simulink model "bike_model_pidTuning"  (R2018b)
settings: Solver=FixedStepAuto  StartTime=0.0  StopTime=sim_time  FixedStep=Ts_IMU  MaxStep=Ts  RelTol=1e-3
values from neighbouring files (symbols this model uses):
  a_compFilter = b_compFilter - 0.77    (= 0.325)    [configuration.m]    (also in configuration_boxMovedCenter.m = 0.4964; configuration_pidTuning.m)
  b_compFilter = 1.095    [configuration.m]    (also in configuration_boxMovedCenter.m; configuration_pidTuning.m)
  b_real = 1.095    [configuration.m]    (also in configuration_boxMovedCenter.m; configuration_pidTuning.m)
  direct_control = 1    [configuration.m]    (also in configuration_boxMovedCenter.m; configuration_pidTuning.m)
  g = 9.81    [configuration.m]    (also in configuration_boxMovedCenter.m; configuration_pidTuning.m; positionEstimation.m = 9.82)
  IMU_height_real = 0.45    [configuration.m]    (also in configuration_boxMovedCenter.m; configuration_pidTuning.m)
  initial_states = [deg2rad(2) deg2rad(0) deg2rad(0)]    [configuration.m]    (also in configuration_boxMovedCenter.m = [deg2rad(5) deg2rad(-2) deg2rad(0)]; configuration_pidTuning.m = [deg2rad(0) deg2rad(0) deg2rad(0)])
  initial_x = x_ini_diff    (= 0)    [paths.m]
  initial_y = y_ini_diff    (= 0)    [paths.m]
  input_velocity = 3    [configuration.m]    (also in configuration_boxMovedCenter.m; configuration_pidTuning.m)
  K_dir = [0.2 0 0]    [tuning_pid.m]
  K_PID = K_comparison(index,:)    [tuning_pid.m]
  lambda_compFilter = deg2rad(70)    [configuration.m]    (also in configuration_boxMovedCenter.m; configuration_pidTuning.m)
  lambda_real = deg2rad(70)    [configuration.m]    (also in configuration_boxMovedCenter.m; configuration_pidTuning.m)
  look_ahead = 0    [configuration.m]    (also in configuration_boxMovedCenter.m; configuration_pidTuning.m)
  parameters_compFilter = [g h_compFilter b_compFilter a_compFilter lambda_compFilter c_compFilter]    [configuration.m]    (also in configuration_boxMovedCenter.m; configuration_pidTuning.m)
  parameters_f_b_real = [m_frame_real m_box_real h_frame_real h_box_real a_frame_real a_box_real c_frame_real c_box_real b_frame_real b_box_real l_frame_real l_box_real]    [configuration.m]    (also in configuration_boxMovedCenter.m; configuration_pidTuning.m)
  parameters_real = [g h_real b_real a_real lambda_real c_real]    [configuration.m]    (also in configuration_boxMovedCenter.m; configuration_pidTuning.m)
  path_x = [path_x1 path_x2 path_x3 path_x4 path_x5]    [paths.m]
  path_y = [path_y1 path_y2 path_y3 path_y4 path_y5]    [paths.m]
  plant_model = 1    [configuration.m]    (also in configuration_boxMovedCenter.m; configuration_pidTuning.m)
  Ts = 0.04    [configuration.m]    (also in configuration_boxMovedCenter.m; configuration_pidTuning.m; positionEstimation.m)
  Ts_IMU = 0.04    [configuration.m]    (also in configuration_boxMovedCenter.m; configuration_pidTuning.m)
undefined symbols (not defined in the file or in its folder): A, B, cumulative_dist_along_path, curvature, DiscIntNeverNeededParam, lqr_gains, sys_con, sys_dis, velocity_lqr
libraries: simulink x23, dspsigops x2
(part 2 of 3)

== system bike_model_pidTuning/Path Tracking Controller PID Tuning 2/Tuning of Direction (Heading Control) ==
  Step input : Inport
  Estimated Heading : Inport  Port=2
  Discrete-Time Integrator : DiscreteIntegrator  Commented=on  SampleTime=-1  ICPrevOutput=DiscIntNeverNeededParam  ICPrevScaledInput=DiscIntNeverNeededParam
  Gain1 : Gain  Commented=on  Gain=sin(lambda_compFilter)
  Measured Bike Angles to Global Angles : Subsystem  Commented=on
  Measured Global Angles to Global Coordinates : Subsystem  Commented=on
  PID Control Direction2 : simulink/Continuous/PID Controller  Controller=PID  Form=Parallel  TimeDomain=Discrete-time  SampleTime=Ts  IntegratorMethod=Forward Euler  FilterMethod=Forward Euler  ControllerParametersSource=internal  P=K_PID(1)  I=K_PID(2)  D=K_PID(3)  UseFilter=off  N=100  TunerSelectOption=Transfer Function Based (PID Tuner App)  InitialConditionSource=internal  InitialConditionForIntegrator=0  InitialConditionForFilter=0  DifferentiatorICPrevScaledInput=0  ExternalReset=none  TrackingMode=off  Kt=1  LimitOutput=off  UpperSaturationLimit=inf  LowerSaturationLimit=-inf  LinearizeAsGain=on  AntiWindupMode=none  Kb=1  POutMin=[]  POutMax=[]  IOutMin=[]  IOutMax=[]  DOutMin=[]  DOutMax=[]  NOutMin=[]  NOutMax=[]  SumOutMin=[]  SumOutMax=[]  SaturationOutMin=[]  SaturationOutMax=[]  PParamMin=[]  PParamMax=[]  IParamMin=[]  IParamMax=[]  DParamMin=[]  DParamMax=[]  NParamMin=[]  NParamMax=[]  KbParamMin=[]  KbParamMax=[]  KtParamMin=[]  KtParamMax=[]  KbOutMin=[]  KbOutMax=[]  KtOutMin=[]  KtOutMax=[]  IntegratorOutMin=[]  IntegratorOutMax=[]  FilterOutMin=[]  FilterOutMax=[]  SumI1OutMin=[]  SumI1OutMax=[]  SumI2OutMin=[]  SumI2OutMax=[]  SumI3OutMin=[]  SumI3OutMax=[]  SumI4OutMin=[]  SumI4OutMax=[]  SumDOutMin=[]  SumDOutMax=[]  DifferentiatorOutMin=[]  DifferentiatorOutMax=[]  FilterDiffOutCoefMin=[]  FilterDiffOutCoefMax=[]  ReciprocalOutMin=[]  ReciprocalOutMax=[]  SumDenOutMin=[]  SumDenOutMax=[]  SumNumOutMin=[]  SumNumOutMax=[]  DivideOutMin=[]  DivideOutMax=[]  IntegratorContinuousStateAttributes=''  IntegratorStateMustResolveToSignalObject=off  IntegratorRTWStateStorageClass=Auto  FilterContinuousStateAttributes=''  FilterStateMustResolveToSignalObject=off  FilterRTWStateStorageClass=Auto  ParallelPVariant=InternalParameters  IdealPVariant=Disabled  IVariant=InternalParameters  DVariant=InternalParameters  IntegratorVariant=Discrete  SatVariant=Disabled  AWVariant=Passthrough  PCopyVariant=Disabled  TRVariant=Disabled  FdbkBlocksVariant=Forward  IdealPFdbkVariant=Disabled  SatFdbkVariant=Disabled  DerivativeFilterVariant=Differentiator  NVariant=Passthrough  NCopyVariant=Disabled_SignalSpec  FilterICVariant=InternalICsDifferentiator  IntegratorICVariant=InternalICs  ExternalResetVariant=Disabled  TRSumVariant=Passthrough  SumFdbkVariant=Disabled  SumVariant=Sum_PID
  Psi to Delta : Subsystem  Commented=on
  Sum : Sum  Commented=on  Inputs=++|
  Sum4 : Sum  Inputs=+--
  To Workspace5 : ToWorkspace  Commented=on  VariableName=pos_vel_int1  SaveFormat=Timeseries  SampleTime=-1
  Steering Reference : Outport
  Controlled Output : Outport  Port=2
  wires:
  Estimated Heading/1 -> Controlled Output/1, Sum4/3
  Sum4/1 -> PID Control Direction2/1  "Delta Reference = Psi Sigma - Nu"
  Step input/1 -> Sum4/1
  PID Control Direction2/1 -> Steering Reference/1
  Measured Bike Angles to Global Angles/1(Psi) -> Sum/2, Measured Global Angles to Global Coordinates/2(Psi)
  ? -> Gain1/1
  Measured Global Angles to Global Coordinates/1("Velocity (Xdot, Ydot)") -> Discrete-Time Integrator/1
  Gain1/1 -> Measured Bike Angles to Global Angles/2(Measured Steering Angle)
  Sum/1 -> ?
  ? -> Measured Bike Angles to Global Angles/1(Velocity), Measured Global Angles to Global Coordinates/1(Velocity)
  Measured Bike Angles to Global Angles/2(Beta) -> Measured Global Angles to Global Coordinates/3(Beta), Sum/1
  Discrete-Time Integrator/1 -> To Workspace5/1

== system bike_model_pidTuning/Path Tracking Controller PID Tuning 2/Tuning of Direction (Heading Control)2 ==
  Step input : Inport
  Measured Steering : Inport  Port=2
  PID Control Direction2 : simulink/Continuous/PID Controller  Controller=PI  Form=Parallel  TimeDomain=Discrete-time  SampleTime=Ts  IntegratorMethod=Forward Euler  FilterMethod=Forward Euler  ControllerParametersSource=internal  P=0.578359413467721  I=0.617399561418389  D=0  UseFilter=on  N=100  TunerSelectOption=Transfer Function Based (PID Tuner App)  InitialConditionSource=internal  InitialConditionForIntegrator=0  InitialConditionForFilter=0  DifferentiatorICPrevScaledInput=0  ExternalReset=none  TrackingMode=off  Kt=1  LimitOutput=off  UpperSaturationLimit=inf  LowerSaturationLimit=-inf  LinearizeAsGain=on  AntiWindupMode=none  Kb=1  POutMin=[]  POutMax=[]  IOutMin=[]  IOutMax=[]  DOutMin=[]  DOutMax=[]  NOutMin=[]  NOutMax=[]  SumOutMin=[]  SumOutMax=[]  SaturationOutMin=[]  SaturationOutMax=[]  PParamMin=[]  PParamMax=[]  IParamMin=[]  IParamMax=[]  DParamMin=[]  DParamMax=[]  NParamMin=[]  NParamMax=[]  KbParamMin=[]  KbParamMax=[]  KtParamMin=[]  KtParamMax=[]  KbOutMin=[]  KbOutMax=[]  KtOutMin=[]  KtOutMax=[]  IntegratorOutMin=[]  IntegratorOutMax=[]  FilterOutMin=[]  FilterOutMax=[]  SumI1OutMin=[]  SumI1OutMax=[]  SumI2OutMin=[]  SumI2OutMax=[]  SumI3OutMin=[]  SumI3OutMax=[]  SumI4OutMin=[]  SumI4OutMax=[]  SumDOutMin=[]  SumDOutMax=[]  DifferentiatorOutMin=[]  DifferentiatorOutMax=[]  FilterDiffOutCoefMin=[]  FilterDiffOutCoefMax=[]  ReciprocalOutMin=[]  ReciprocalOutMax=[]  SumDenOutMin=[]  SumDenOutMax=[]  SumNumOutMin=[]  SumNumOutMax=[]  DivideOutMin=[]  DivideOutMax=[]  IntegratorContinuousStateAttributes=''  IntegratorStateMustResolveToSignalObject=off  IntegratorRTWStateStorageClass=Auto  FilterContinuousStateAttributes=''  FilterStateMustResolveToSignalObject=off  FilterRTWStateStorageClass=Auto  ParallelPVariant=InternalParameters  IdealPVariant=Disabled  IVariant=InternalParameters  DVariant=Disabled  IntegratorVariant=Discrete  SatVariant=Disabled  AWVariant=Passthrough  PCopyVariant=Disabled  TRVariant=Disabled  FdbkBlocksVariant=Forward  IdealPFdbkVariant=Disabled  SatFdbkVariant=Disabled  DerivativeFilterVariant=Disabled  NVariant=Disabled  NCopyVariant=Disabled_SignalSpec  FilterICVariant=Disabled  IntegratorICVariant=InternalICs  ExternalResetVariant=Disabled  TRSumVariant=Passthrough  SumFdbkVariant=Disabled  SumVariant=Sum_PI
  Sum4 : Sum  Inputs=+--
  Transfer Fcn : TransferFcn  Numerator=[1 0]  Denominator=[a_compFilter/b_compFilter input_velocity/a_compFilter]
  Steering Reference : Outport
  Controlled Output : Outport  Port=2
  wires:
  Step input/1 -> Transfer Fcn/1
  PID Control Direction2/1 -> Steering Reference/1
  Measured Steering/1 -> Controlled Output/1, Sum4/3
  Transfer Fcn/1 -> Sum4/1
  Sum4/1 -> PID Control Direction2/1

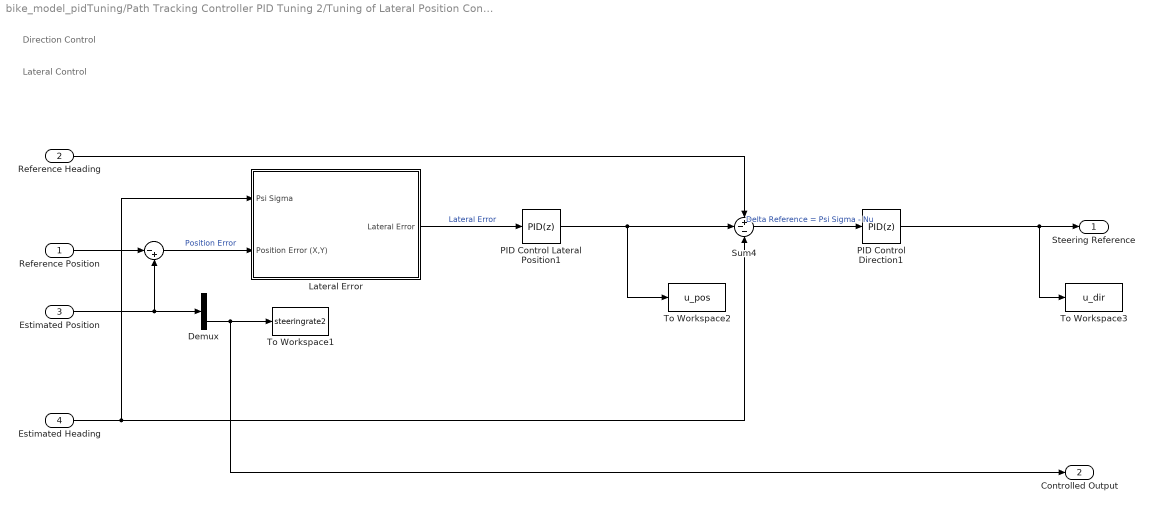
== system bike_model_pidTuning/Path Tracking Controller PID Tuning 2/Tuning of Lateral Position Control ==
  note: Direction Control
  note: Lateral Control
  Reference Position : Inport
  Reference Heading : Inport  Port=2
  Estimated Position : Inport  Port=3
  Estimated Heading : Inport  Port=4
  " " : Sum  Inputs=|-+
  Demux : Demux  Outputs=2
  Lateral Error : Subsystem  SystemSampleTime=Ts
  PID Control Lateral Position1 : simulink/Continuous/PID Controller  Controller=PID  Form=Parallel  TimeDomain=Discrete-time  SampleTime=Ts  IntegratorMethod=Forward Euler  FilterMethod=Forward Euler  ControllerParametersSource=internal  P=K_PID(1)  I=K_PID(2)  D=K_PID(3)  UseFilter=off  N=38.085941813801  TunerSelectOption=Transfer Function Based (PID Tuner App)  InitialConditionSource=internal  InitialConditionForIntegrator=0  InitialConditionForFilter=0  DifferentiatorICPrevScaledInput=0  ExternalReset=none  TrackingMode=off  Kt=1  LimitOutput=off  UpperSaturationLimit=inf  LowerSaturationLimit=-inf  LinearizeAsGain=on  AntiWindupMode=none  Kb=1  POutMin=[]  POutMax=[]  IOutMin=[]  IOutMax=[]  DOutMin=[]  DOutMax=[]  NOutMin=[]  NOutMax=[]  SumOutMin=[]  SumOutMax=[]  SaturationOutMin=[]  SaturationOutMax=[]  PParamMin=[]  PParamMax=[]  IParamMin=[]  IParamMax=[]  DParamMin=[]  DParamMax=[]  NParamMin=[]  NParamMax=[]  KbParamMin=[]  KbParamMax=[]  KtParamMin=[]  KtParamMax=[]  KbOutMin=[]  KbOutMax=[]  KtOutMin=[]  KtOutMax=[]  IntegratorOutMin=[]  IntegratorOutMax=[]  FilterOutMin=[]  FilterOutMax=[]  SumI1OutMin=[]  SumI1OutMax=[]  SumI2OutMin=[]  SumI2OutMax=[]  SumI3OutMin=[]  SumI3OutMax=[]  SumI4OutMin=[]  SumI4OutMax=[]  SumDOutMin=[]  SumDOutMax=[]  DifferentiatorOutMin=[]  DifferentiatorOutMax=[]  FilterDiffOutCoefMin=[]  FilterDiffOutCoefMax=[]  ReciprocalOutMin=[]  ReciprocalOutMax=[]  SumDenOutMin=[]  SumDenOutMax=[]  SumNumOutMin=[]  SumNumOutMax=[]  DivideOutMin=[]  DivideOutMax=[]  IntegratorContinuousStateAttributes=''  IntegratorStateMustResolveToSignalObject=off  IntegratorRTWStateStorageClass=Auto  FilterContinuousStateAttributes=''  FilterStateMustResolveToSignalObject=off  FilterRTWStateStorageClass=Auto  ParallelPVariant=InternalParameters  IdealPVariant=Disabled  IVariant=InternalParameters  DVariant=InternalParameters  IntegratorVariant=Discrete  SatVariant=Disabled  AWVariant=Passthrough  PCopyVariant=Disabled  TRVariant=Disabled  FdbkBlocksVariant=Forward  IdealPFdbkVariant=Disabled  SatFdbkVariant=Disabled  DerivativeFilterVariant=Differentiator  NVariant=Passthrough  NCopyVariant=Disabled_SignalSpec  FilterICVariant=InternalICsDifferentiator  IntegratorICVariant=InternalICs  ExternalResetVariant=Disabled  TRSumVariant=Passthrough  SumFdbkVariant=Disabled  SumVariant=Sum_PID
  PID Control Direction1 : simulink/Continuous/PID Controller  Controller=PID  Form=Parallel  TimeDomain=Discrete-time  SampleTime=Ts  IntegratorMethod=Forward Euler  FilterMethod=Forward Euler  ControllerParametersSource=internal  P=K_dir(1)  I=K_dir(2)  D=K_dir(3)  UseFilter=off  N=100  TunerSelectOption=Transfer Function Based (PID Tuner App)  InitialConditionSource=internal  InitialConditionForIntegrator=0  InitialConditionForFilter=0  DifferentiatorICPrevScaledInput=0  ExternalReset=none  TrackingMode=off  Kt=1  LimitOutput=off  UpperSaturationLimit=inf  LowerSaturationLimit=-inf  LinearizeAsGain=on  AntiWindupMode=none  Kb=1  POutMin=[]  POutMax=[]  IOutMin=[]  IOutMax=[]  DOutMin=[]  DOutMax=[]  NOutMin=[]  NOutMax=[]  SumOutMin=[]  SumOutMax=[]  SaturationOutMin=[]  SaturationOutMax=[]  PParamMin=[]  PParamMax=[]  IParamMin=[]  IParamMax=[]  DParamMin=[]  DParamMax=[]  NParamMin=[]  NParamMax=[]  KbParamMin=[]  KbParamMax=[]  KtParamMin=[]  KtParamMax=[]  KbOutMin=[]  KbOutMax=[]  KtOutMin=[]  KtOutMax=[]  IntegratorOutMin=[]  IntegratorOutMax=[]  FilterOutMin=[]  FilterOutMax=[]  SumI1OutMin=[]  SumI1OutMax=[]  SumI2OutMin=[]  SumI2OutMax=[]  SumI3OutMin=[]  SumI3OutMax=[]  SumI4OutMin=[]  SumI4OutMax=[]  SumDOutMin=[]  SumDOutMax=[]  DifferentiatorOutMin=[]  DifferentiatorOutMax=[]  FilterDiffOutCoefMin=[]  FilterDiffOutCoefMax=[]  ReciprocalOutMin=[]  ReciprocalOutMax=[]  SumDenOutMin=[]  SumDenOutMax=[]  SumNumOutMin=[]  SumNumOutMax=[]  DivideOutMin=[]  DivideOutMax=[]  IntegratorContinuousStateAttributes=''  IntegratorStateMustResolveToSignalObject=off  IntegratorRTWStateStorageClass=Auto  FilterContinuousStateAttributes=''  FilterStateMustResolveToSignalObject=off  FilterRTWStateStorageClass=Auto  ParallelPVariant=InternalParameters  IdealPVariant=Disabled  IVariant=InternalParameters  DVariant=InternalParameters  IntegratorVariant=Discrete  SatVariant=Disabled  AWVariant=Passthrough  PCopyVariant=Disabled  TRVariant=Disabled  FdbkBlocksVariant=Forward  IdealPFdbkVariant=Disabled  SatFdbkVariant=Disabled  DerivativeFilterVariant=Differentiator  NVariant=Passthrough  NCopyVariant=Disabled_SignalSpec  FilterICVariant=InternalICsDifferentiator  IntegratorICVariant=InternalICs  ExternalResetVariant=Disabled  TRSumVariant=Passthrough  SumFdbkVariant=Disabled  SumVariant=Sum_PID
  Sum4 : Sum  Inputs=+--
  To Workspace1 : ToWorkspace  VariableName=steeringrate2  SaveFormat=Timeseries  SampleTime=Ts
  To Workspace2 : ToWorkspace  VariableName=u_pos  SaveFormat=Timeseries  SampleTime=Ts
  To Workspace3 : ToWorkspace  VariableName=u_dir  SaveFormat=Timeseries  SampleTime=Ts
  Steering Reference : Outport
  Controlled Output : Outport  Port=2
  wires:
  PID Control Lateral Position1/1 -> To Workspace2/1, Sum4/2
  Reference Heading/1 -> Sum4/1
  Lateral Error/1(Lateral Error) -> PID Control Lateral Position1/1  "Lateral Error"
  Reference Position/1 -> " "/1
  Estimated Heading/1 -> Lateral Error/1(Psi Sigma), Sum4/3
  " "/1 -> Lateral Error/2(Position Error (X,Y))  "Position Error"
  Sum4/1 -> PID Control Direction1/1  "Delta Reference = Psi Sigma - Nu"
  Demux/2 -> Controlled Output/1, To Workspace1/1
  PID Control Direction1/1 -> To Workspace3/1, Steering Reference/1
  Estimated Position/1 -> " "/2, Demux/1

== system bike_model_pidTuning/Path Tracking Controller PID Tuning 2/Tuning of Lateral Position Control1 ==
  note: Direction Control
  note: Lateral Control
  Reference Position : Inport
  Reference Heading : Inport  Port=2
  Estimated Position : Inport  Port=3
  Estimated Heading : Inport  Port=4
  " " : Sum  Inputs=|-+
  Demux : Demux  Outputs=2
  Lateral Error : Subsystem  SystemSampleTime=Ts
  PID Control Lateral Position : simulink/Continuous/PID Controller  Controller=PID  Form=Parallel  TimeDomain=Discrete-time  SampleTime=Ts  IntegratorMethod=Forward Euler  FilterMethod=Forward Euler  ControllerParametersSource=internal  P=0.0553  I=0.000972  D=0.699  UseFilter=on  N=100  TunerSelectOption=Transfer Function Based (PID Tuner App)  InitialConditionSource=internal  InitialConditionForIntegrator=0  InitialConditionForFilter=0  DifferentiatorICPrevScaledInput=0  ExternalReset=none  TrackingMode=off  Kt=1  LimitOutput=off  UpperSaturationLimit=inf  LowerSaturationLimit=-inf  LinearizeAsGain=on  AntiWindupMode=none  Kb=1  POutMin=[]  POutMax=[]  IOutMin=[]  IOutMax=[]  DOutMin=[]  DOutMax=[]  NOutMin=[]  NOutMax=[]  SumOutMin=[]  SumOutMax=[]  SaturationOutMin=[]  SaturationOutMax=[]  PParamMin=[]  PParamMax=[]  IParamMin=[]  IParamMax=[]  DParamMin=[]  DParamMax=[]  NParamMin=[]  NParamMax=[]  KbParamMin=[]  KbParamMax=[]  KtParamMin=[]  KtParamMax=[]  KbOutMin=[]  KbOutMax=[]  KtOutMin=[]  KtOutMax=[]  IntegratorOutMin=[]  IntegratorOutMax=[]  FilterOutMin=[]  FilterOutMax=[]  SumI1OutMin=[]  SumI1OutMax=[]  SumI2OutMin=[]  SumI2OutMax=[]  SumI3OutMin=[]  SumI3OutMax=[]  SumI4OutMin=[]  SumI4OutMax=[]  SumDOutMin=[]  SumDOutMax=[]  DifferentiatorOutMin=[]  DifferentiatorOutMax=[]  FilterDiffOutCoefMin=[]  FilterDiffOutCoefMax=[]  ReciprocalOutMin=[]  ReciprocalOutMax=[]  SumDenOutMin=[]  SumDenOutMax=[]  SumNumOutMin=[]  SumNumOutMax=[]  DivideOutMin=[]  DivideOutMax=[]  IntegratorContinuousStateAttributes=''  IntegratorStateMustResolveToSignalObject=off  IntegratorRTWStateStorageClass=Auto  FilterContinuousStateAttributes=''  FilterStateMustResolveToSignalObject=off  FilterRTWStateStorageClass=Auto  ParallelPVariant=InternalParameters  IdealPVariant=Disabled  IVariant=InternalParameters  DVariant=InternalParameters  IntegratorVariant=Discrete  SatVariant=Disabled  AWVariant=Passthrough  PCopyVariant=Disabled  TRVariant=Disabled  FdbkBlocksVariant=Forward  IdealPFdbkVariant=Disabled  SatFdbkVariant=Disabled  DerivativeFilterVariant=ForwardEulerFilter  NVariant=InternalParameters  NCopyVariant=Disabled  FilterICVariant=InternalICsFilter  IntegratorICVariant=InternalICs  ExternalResetVariant=Disabled  TRSumVariant=Passthrough  SumFdbkVariant=Disabled  SumVariant=Sum_PID
  PID Control Direction2 : simulink/Continuous/PID Controller  Controller=PI  Form=Parallel  TimeDomain=Discrete-time  SampleTime=Ts  IntegratorMethod=Forward Euler  FilterMethod=Forward Euler  ControllerParametersSource=internal  P=0.578359413467721  I=0.617399561418389  D=0  UseFilter=on  N=100  TunerSelectOption=Transfer Function Based (PID Tuner App)  InitialConditionSource=internal  InitialConditionForIntegrator=0  InitialConditionForFilter=0  DifferentiatorICPrevScaledInput=0  ExternalReset=none  TrackingMode=off  Kt=1  LimitOutput=off  UpperSaturationLimit=inf  LowerSaturationLimit=-inf  LinearizeAsGain=on  AntiWindupMode=none  Kb=1  POutMin=[]  POutMax=[]  IOutMin=[]  IOutMax=[]  DOutMin=[]  DOutMax=[]  NOutMin=[]  NOutMax=[]  SumOutMin=[]  SumOutMax=[]  SaturationOutMin=[]  SaturationOutMax=[]  PParamMin=[]  PParamMax=[]  IParamMin=[]  IParamMax=[]  DParamMin=[]  DParamMax=[]  NParamMin=[]  NParamMax=[]  KbParamMin=[]  KbParamMax=[]  KtParamMin=[]  KtParamMax=[]  KbOutMin=[]  KbOutMax=[]  KtOutMin=[]  KtOutMax=[]  IntegratorOutMin=[]  IntegratorOutMax=[]  FilterOutMin=[]  FilterOutMax=[]  SumI1OutMin=[]  SumI1OutMax=[]  SumI2OutMin=[]  SumI2OutMax=[]  SumI3OutMin=[]  SumI3OutMax=[]  SumI4OutMin=[]  SumI4OutMax=[]  SumDOutMin=[]  SumDOutMax=[]  DifferentiatorOutMin=[]  DifferentiatorOutMax=[]  FilterDiffOutCoefMin=[]  FilterDiffOutCoefMax=[]  ReciprocalOutMin=[]  ReciprocalOutMax=[]  SumDenOutMin=[]  SumDenOutMax=[]  SumNumOutMin=[]  SumNumOutMax=[]  DivideOutMin=[]  DivideOutMax=[]  IntegratorContinuousStateAttributes=''  IntegratorStateMustResolveToSignalObject=off  IntegratorRTWStateStorageClass=Auto  FilterContinuousStateAttributes=''  FilterStateMustResolveToSignalObject=off  FilterRTWStateStorageClass=Auto  ParallelPVariant=InternalParameters  IdealPVariant=Disabled  IVariant=InternalParameters  DVariant=Disabled  IntegratorVariant=Discrete  SatVariant=Disabled  AWVariant=Passthrough  PCopyVariant=Disabled  TRVariant=Disabled  FdbkBlocksVariant=Forward  IdealPFdbkVariant=Disabled  SatFdbkVariant=Disabled  DerivativeFilterVariant=Disabled  NVariant=Disabled  NCopyVariant=Disabled_SignalSpec  FilterICVariant=Disabled  IntegratorICVariant=InternalICs  ExternalResetVariant=Disabled  TRSumVariant=Passthrough  SumFdbkVariant=Disabled  SumVariant=Sum_PI
  Sum4 : Sum  Inputs=+--
  Transfer Fcn : TransferFcn  Numerator=[1 0]  Denominator=[a_compFilter/b_compFilter input_velocity/a_compFilter]
  Steering Reference : Outport
  Controlled Output : Outport  Port=2
  wires:
  Reference Heading/1 -> Transfer Fcn/1, Lateral Error/1(Psi Sigma)
  Lateral Error/1(Lateral Error) -> PID Control Lateral Position/1  "Lateral Error"
  Reference Position/1 -> " "/1
  Estimated Heading/1 -> Sum4/3
  " "/1 -> Lateral Error/2(Position Error (X,Y))  "Position Error"
  Sum4/1 -> PID Control Direction2/1  "Delta Reference = Psi Sigma - Nu"
  Demux/2 -> Controlled Output/1
  PID Control Direction2/1 -> Steering Reference/1
  Estimated Position/1 -> " "/2, Demux/1
  Transfer Fcn/1 -> Sum4/1
  PID Control Lateral Position/1 -> Sum4/2

== system bike_model_pidTuning/Path Tracking Controller PID Tuning1/Step response of the system ==
  Step input : Inport
  Measured Steering Angle : Inport  Port=2
  Gain : Gain  Gain=2/3
  Steering Reference : Outport
  Controlled Output : Outport  Port=2
  wires:
  Step input/1 -> Gain/1
  Measured Steering Angle/1 -> Controlled Output/1
  Gain/1 -> Steering Reference/1

== system bike_model_pidTuning/Path Tracking Controller PID Tuning1/Tuning of Direction (Heading Control) ==
  Step input : Inport
  Estimated Heading : Inport  Port=2
  Measured Steering Angle : Inport  Port=3
  Gain1 : Gain  Gain=1%sin(lambda_real)
  PID Control Direction : simulink/Continuous/PID Controller  Controller=PI  Form=Parallel  TimeDomain=Discrete-time  SampleTime=Ts  IntegratorMethod=Forward Euler  FilterMethod=Forward Euler  ControllerParametersSource=internal  P=0.0712859744206787*2  I=0.000227125326188444/2  D=0  UseFilter=on  N=100  TunerSelectOption=Transfer Function Based (PID Tuner App)  InitialConditionSource=internal  InitialConditionForIntegrator=0  InitialConditionForFilter=0  DifferentiatorICPrevScaledInput=0  ExternalReset=none  TrackingMode=off  Kt=1  LimitOutput=off  UpperSaturationLimit=inf  LowerSaturationLimit=-inf  LinearizeAsGain=on  AntiWindupMode=none  Kb=1  POutMin=[]  POutMax=[]  IOutMin=[]  IOutMax=[]  DOutMin=[]  DOutMax=[]  NOutMin=[]  NOutMax=[]  SumOutMin=[]  SumOutMax=[]  SaturationOutMin=[]  SaturationOutMax=[]  PParamMin=[]  PParamMax=[]  IParamMin=[]  IParamMax=[]  DParamMin=[]  DParamMax=[]  NParamMin=[]  NParamMax=[]  KbParamMin=[]  KbParamMax=[]  KtParamMin=[]  KtParamMax=[]  KbOutMin=[]  KbOutMax=[]  KtOutMin=[]  KtOutMax=[]  IntegratorOutMin=[]  IntegratorOutMax=[]  FilterOutMin=[]  FilterOutMax=[]  SumI1OutMin=[]  SumI1OutMax=[]  SumI2OutMin=[]  SumI2OutMax=[]  SumI3OutMin=[]  SumI3OutMax=[]  SumI4OutMin=[]  SumI4OutMax=[]  SumDOutMin=[]  SumDOutMax=[]  DifferentiatorOutMin=[]  DifferentiatorOutMax=[]  FilterDiffOutCoefMin=[]  FilterDiffOutCoefMax=[]  ReciprocalOutMin=[]  ReciprocalOutMax=[]  SumDenOutMin=[]  SumDenOutMax=[]  SumNumOutMin=[]  SumNumOutMax=[]  DivideOutMin=[]  DivideOutMax=[]  IntegratorContinuousStateAttributes=''  IntegratorStateMustResolveToSignalObject=off  IntegratorRTWStateStorageClass=Auto  FilterContinuousStateAttributes=''  FilterStateMustResolveToSignalObject=off  FilterRTWStateStorageClass=Auto  ParallelPVariant=InternalParameters  IdealPVariant=Disabled  IVariant=InternalParameters  DVariant=Disabled  IntegratorVariant=Discrete  SatVariant=Disabled  AWVariant=Passthrough  PCopyVariant=Disabled  TRVariant=Disabled  FdbkBlocksVariant=Forward  IdealPFdbkVariant=Disabled  SatFdbkVariant=Disabled  DerivativeFilterVariant=Disabled  NVariant=Disabled  NCopyVariant=Disabled_SignalSpec  FilterICVariant=Disabled  IntegratorICVariant=InternalICs  ExternalResetVariant=Disabled  TRSumVariant=Passthrough  SumFdbkVariant=Disabled  SumVariant=Sum_PI
  PID Control Steering : simulink/Continuous/PID Controller  Controller=PI  Form=Parallel  TimeDomain=Discrete-time  SampleTime=Ts  IntegratorMethod=Forward Euler  FilterMethod=Forward Euler  ControllerParametersSource=internal  P=0.219020351848633  I=0.4510120195392  D=0  UseFilter=on  N=100  TunerSelectOption=Transfer Function Based (PID Tuner App)  InitialConditionSource=internal  InitialConditionForIntegrator=0  InitialConditionForFilter=0  DifferentiatorICPrevScaledInput=0  ExternalReset=none  TrackingMode=off  Kt=1  LimitOutput=off  UpperSaturationLimit=inf  LowerSaturationLimit=-inf  LinearizeAsGain=on  AntiWindupMode=none  Kb=1  POutMin=[]  POutMax=[]  IOutMin=[]  IOutMax=[]  DOutMin=[]  DOutMax=[]  NOutMin=[]  NOutMax=[]  SumOutMin=[]  SumOutMax=[]  SaturationOutMin=[]  SaturationOutMax=[]  PParamMin=[]  PParamMax=[]  IParamMin=[]  IParamMax=[]  DParamMin=[]  DParamMax=[]  NParamMin=[]  NParamMax=[]  KbParamMin=[]  KbParamMax=[]  KtParamMin=[]  KtParamMax=[]  KbOutMin=[]  KbOutMax=[]  KtOutMin=[]  KtOutMax=[]  IntegratorOutMin=[]  IntegratorOutMax=[]  FilterOutMin=[]  FilterOutMax=[]  SumI1OutMin=[]  SumI1OutMax=[]  SumI2OutMin=[]  SumI2OutMax=[]  SumI3OutMin=[]  SumI3OutMax=[]  SumI4OutMin=[]  SumI4OutMax=[]  SumDOutMin=[]  SumDOutMax=[]  DifferentiatorOutMin=[]  DifferentiatorOutMax=[]  FilterDiffOutCoefMin=[]  FilterDiffOutCoefMax=[]  ReciprocalOutMin=[]  ReciprocalOutMax=[]  SumDenOutMin=[]  SumDenOutMax=[]  SumNumOutMin=[]  SumNumOutMax=[]  DivideOutMin=[]  DivideOutMax=[]  IntegratorContinuousStateAttributes=''  IntegratorStateMustResolveToSignalObject=off  IntegratorRTWStateStorageClass=Auto  FilterContinuousStateAttributes=''  FilterStateMustResolveToSignalObject=off  FilterRTWStateStorageClass=Auto  ParallelPVariant=InternalParameters  IdealPVariant=Disabled  IVariant=InternalParameters  DVariant=Disabled  IntegratorVariant=Discrete  SatVariant=Disabled  AWVariant=Passthrough  PCopyVariant=Disabled  TRVariant=Disabled  FdbkBlocksVariant=Forward  IdealPFdbkVariant=Disabled  SatFdbkVariant=Disabled  DerivativeFilterVariant=Disabled  NVariant=Disabled  NCopyVariant=Disabled_SignalSpec  FilterICVariant=Disabled  IntegratorICVariant=InternalICs  ExternalResetVariant=Disabled  TRSumVariant=Passthrough  SumFdbkVariant=Disabled  SumVariant=Sum_PI
  Sum1 : Sum  Inputs=|+-
  Sum4 : Sum  Inputs=+--
  Steering Reference : Outport
  Controlled Output : Outport  Port=2
  wires:
  Sum1/1 -> PID Control Steering/1  "Delta Error"
  PID Control Direction/1 -> Sum1/1
  Estimated Heading/1 -> Sum4/3, Controlled Output/1
  Sum4/1 -> PID Control Direction/1  "Delta Reference = Psi Sigma - Nu"
  Step input/1 -> Sum4/1
  Measured Steering Angle/1 -> Gain1/1
  Gain1/1 -> Sum1/2
  PID Control Steering/1 -> Steering Reference/1

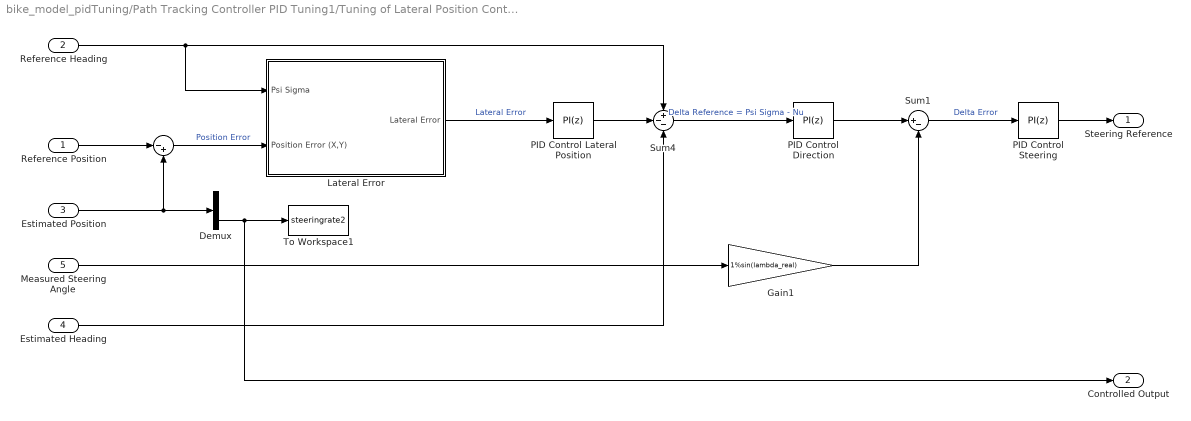
== system bike_model_pidTuning/Path Tracking Controller PID Tuning1/Tuning of Lateral Position Control ==
  Reference Position : Inport
  Reference Heading : Inport  Port=2
  Estimated Position : Inport  Port=3
  Estimated Heading : Inport  Port=4
  Measured Steering Angle : Inport  Port=5
  " " : Sum  Inputs=|-+
  Demux : Demux  Outputs=2
  Gain1 : Gain  Gain=1%sin(lambda_real)
  Lateral Error : Subsystem  SystemSampleTime=Ts
  PID Control Lateral Position : simulink/Continuous/PID Controller  Controller=PI  Form=Parallel  TimeDomain=Discrete-time  SampleTime=Ts  IntegratorMethod=Forward Euler  FilterMethod=Forward Euler  ControllerParametersSource=internal  P=0.0465435246389258  I=0.000115580509653549  D=0  UseFilter=on  N=100  TunerSelectOption=Transfer Function Based (PID Tuner App)  InitialConditionSource=internal  InitialConditionForIntegrator=0  InitialConditionForFilter=0  DifferentiatorICPrevScaledInput=0  ExternalReset=none  TrackingMode=off  Kt=1  LimitOutput=off  UpperSaturationLimit=inf  LowerSaturationLimit=-inf  LinearizeAsGain=on  AntiWindupMode=none  Kb=1  POutMin=[]  POutMax=[]  IOutMin=[]  IOutMax=[]  DOutMin=[]  DOutMax=[]  NOutMin=[]  NOutMax=[]  SumOutMin=[]  SumOutMax=[]  SaturationOutMin=[]  SaturationOutMax=[]  PParamMin=[]  PParamMax=[]  IParamMin=[]  IParamMax=[]  DParamMin=[]  DParamMax=[]  NParamMin=[]  NParamMax=[]  KbParamMin=[]  KbParamMax=[]  KtParamMin=[]  KtParamMax=[]  KbOutMin=[]  KbOutMax=[]  KtOutMin=[]  KtOutMax=[]  IntegratorOutMin=[]  IntegratorOutMax=[]  FilterOutMin=[]  FilterOutMax=[]  SumI1OutMin=[]  SumI1OutMax=[]  SumI2OutMin=[]  SumI2OutMax=[]  SumI3OutMin=[]  SumI3OutMax=[]  SumI4OutMin=[]  SumI4OutMax=[]  SumDOutMin=[]  SumDOutMax=[]  DifferentiatorOutMin=[]  DifferentiatorOutMax=[]  FilterDiffOutCoefMin=[]  FilterDiffOutCoefMax=[]  ReciprocalOutMin=[]  ReciprocalOutMax=[]  SumDenOutMin=[]  SumDenOutMax=[]  SumNumOutMin=[]  SumNumOutMax=[]  DivideOutMin=[]  DivideOutMax=[]  IntegratorContinuousStateAttributes=''  IntegratorStateMustResolveToSignalObject=off  IntegratorRTWStateStorageClass=Auto  FilterContinuousStateAttributes=''  FilterStateMustResolveToSignalObject=off  FilterRTWStateStorageClass=Auto  ParallelPVariant=InternalParameters  IdealPVariant=Disabled  IVariant=InternalParameters  DVariant=Disabled  IntegratorVariant=Discrete  SatVariant=Disabled  AWVariant=Passthrough  PCopyVariant=Disabled  TRVariant=Disabled  FdbkBlocksVariant=Forward  IdealPFdbkVariant=Disabled  SatFdbkVariant=Disabled  DerivativeFilterVariant=Disabled  NVariant=Disabled  NCopyVariant=Disabled_SignalSpec  FilterICVariant=Disabled  IntegratorICVariant=InternalICs  ExternalResetVariant=Disabled  TRSumVariant=Passthrough  SumFdbkVariant=Disabled  SumVariant=Sum_PI
  PID Control Direction : simulink/Continuous/PID Controller  Controller=PI  Form=Parallel  TimeDomain=Discrete-time  SampleTime=Ts  IntegratorMethod=Forward Euler  FilterMethod=Forward Euler  ControllerParametersSource=internal  P=0.126067479140802  I=0.000739995118675849  D=0  UseFilter=on  N=100  TunerSelectOption=Transfer Function Based (PID Tuner App)  InitialConditionSource=internal  InitialConditionForIntegrator=0  InitialConditionForFilter=0  DifferentiatorICPrevScaledInput=0  ExternalReset=none  TrackingMode=off  Kt=1  LimitOutput=off  UpperSaturationLimit=inf  LowerSaturationLimit=-inf  LinearizeAsGain=on  AntiWindupMode=none  Kb=1  POutMin=[]  POutMax=[]  IOutMin=[]  IOutMax=[]  DOutMin=[]  DOutMax=[]  NOutMin=[]  NOutMax=[]  SumOutMin=[]  SumOutMax=[]  SaturationOutMin=[]  SaturationOutMax=[]  PParamMin=[]  PParamMax=[]  IParamMin=[]  IParamMax=[]  DParamMin=[]  DParamMax=[]  NParamMin=[]  NParamMax=[]  KbParamMin=[]  KbParamMax=[]  KtParamMin=[]  KtParamMax=[]  KbOutMin=[]  KbOutMax=[]  KtOutMin=[]  KtOutMax=[]  IntegratorOutMin=[]  IntegratorOutMax=[]  FilterOutMin=[]  FilterOutMax=[]  SumI1OutMin=[]  SumI1OutMax=[]  SumI2OutMin=[]  SumI2OutMax=[]  SumI3OutMin=[]  SumI3OutMax=[]  SumI4OutMin=[]  SumI4OutMax=[]  SumDOutMin=[]  SumDOutMax=[]  DifferentiatorOutMin=[]  DifferentiatorOutMax=[]  FilterDiffOutCoefMin=[]  FilterDiffOutCoefMax=[]  ReciprocalOutMin=[]  ReciprocalOutMax=[]  SumDenOutMin=[]  SumDenOutMax=[]  SumNumOutMin=[]  SumNumOutMax=[]  DivideOutMin=[]  DivideOutMax=[]  IntegratorContinuousStateAttributes=''  IntegratorStateMustResolveToSignalObject=off  IntegratorRTWStateStorageClass=Auto  FilterContinuousStateAttributes=''  FilterStateMustResolveToSignalObject=off  FilterRTWStateStorageClass=Auto  ParallelPVariant=InternalParameters  IdealPVariant=Disabled  IVariant=InternalParameters  DVariant=Disabled  IntegratorVariant=Discrete  SatVariant=Disabled  AWVariant=Passthrough  PCopyVariant=Disabled  TRVariant=Disabled  FdbkBlocksVariant=Forward  IdealPFdbkVariant=Disabled  SatFdbkVariant=Disabled  DerivativeFilterVariant=Disabled  NVariant=Disabled  NCopyVariant=Disabled_SignalSpec  FilterICVariant=Disabled  IntegratorICVariant=InternalICs  ExternalResetVariant=Disabled  TRSumVariant=Passthrough  SumFdbkVariant=Disabled  SumVariant=Sum_PI
  PID Control Steering : simulink/Continuous/PID Controller  Controller=PI  Form=Parallel  TimeDomain=Discrete-time  SampleTime=Ts  IntegratorMethod=Forward Euler  FilterMethod=Forward Euler  ControllerParametersSource=internal  P=0.219020351848633  I=0.4510120195392  D=0  UseFilter=on  N=100  TunerSelectOption=Transfer Function Based (PID Tuner App)  InitialConditionSource=internal  InitialConditionForIntegrator=0  InitialConditionForFilter=0  DifferentiatorICPrevScaledInput=0  ExternalReset=none  TrackingMode=off  Kt=1  LimitOutput=off  UpperSaturationLimit=inf  LowerSaturationLimit=-inf  LinearizeAsGain=on  AntiWindupMode=none  Kb=1  POutMin=[]  POutMax=[]  IOutMin=[]  IOutMax=[]  DOutMin=[]  DOutMax=[]  NOutMin=[]  NOutMax=[]  SumOutMin=[]  SumOutMax=[]  SaturationOutMin=[]  SaturationOutMax=[]  PParamMin=[]  PParamMax=[]  IParamMin=[]  IParamMax=[]  DParamMin=[]  DParamMax=[]  NParamMin=[]  NParamMax=[]  KbParamMin=[]  KbParamMax=[]  KtParamMin=[]  KtParamMax=[]  KbOutMin=[]  KbOutMax=[]  KtOutMin=[]  KtOutMax=[]  IntegratorOutMin=[]  IntegratorOutMax=[]  FilterOutMin=[]  FilterOutMax=[]  SumI1OutMin=[]  SumI1OutMax=[]  SumI2OutMin=[]  SumI2OutMax=[]  SumI3OutMin=[]  SumI3OutMax=[]  SumI4OutMin=[]  SumI4OutMax=[]  SumDOutMin=[]  SumDOutMax=[]  DifferentiatorOutMin=[]  DifferentiatorOutMax=[]  FilterDiffOutCoefMin=[]  FilterDiffOutCoefMax=[]  ReciprocalOutMin=[]  ReciprocalOutMax=[]  SumDenOutMin=[]  SumDenOutMax=[]  SumNumOutMin=[]  SumNumOutMax=[]  DivideOutMin=[]  DivideOutMax=[]  IntegratorContinuousStateAttributes=''  IntegratorStateMustResolveToSignalObject=off  IntegratorRTWStateStorageClass=Auto  FilterContinuousStateAttributes=''  FilterStateMustResolveToSignalObject=off  FilterRTWStateStorageClass=Auto  ParallelPVariant=InternalParameters  IdealPVariant=Disabled  IVariant=InternalParameters  DVariant=Disabled  IntegratorVariant=Discrete  SatVariant=Disabled  AWVariant=Passthrough  PCopyVariant=Disabled  TRVariant=Disabled  FdbkBlocksVariant=Forward  IdealPFdbkVariant=Disabled  SatFdbkVariant=Disabled  DerivativeFilterVariant=Disabled  NVariant=Disabled  NCopyVariant=Disabled_SignalSpec  FilterICVariant=Disabled  IntegratorICVariant=InternalICs  ExternalResetVariant=Disabled  TRSumVariant=Passthrough  SumFdbkVariant=Disabled  SumVariant=Sum_PI
  Sum1 : Sum  Inputs=|+-
  Sum4 : Sum  Inputs=+--
  To Workspace1 : ToWorkspace  VariableName=steeringrate2  SaveFormat=Timeseries  SampleTime=Ts
  Steering Reference : Outport
  Controlled Output : Outport  Port=2
  wires:
  PID Control Lateral Position/1 -> Sum4/2
  Reference Heading/1 -> Sum4/1, Lateral Error/1(Psi Sigma)
  Sum1/1 -> PID Control Steering/1  "Delta Error"
  PID Control Direction/1 -> Sum1/1
  Gain1/1 -> Sum1/2
  Lateral Error/1(Lateral Error) -> PID Control Lateral Position/1  "Lateral Error"
  Reference Position/1 -> " "/1
  Estimated Heading/1 -> Sum4/3
  " "/1 -> Lateral Error/2(Position Error (X,Y))  "Position Error"
  Sum4/1 -> PID Control Direction/1  "Delta Reference = Psi Sigma - Nu"
  Demux/2 -> Controlled Output/1, To Workspace1/1
  Measured Steering Angle/1 -> Gain1/1
  PID Control Steering/1 -> Steering Reference/1
  Estimated Position/1 -> " "/2, Demux/1

== system bike_model_pidTuning/Path Tracking Controller PID Tuning1/Tuning of Steering Control ==
  Step input : Inport
  Measured Steering Angle : Inport  Port=2
  Gain1 : Gain  Gain=1%sin(lambda_real)
  PID Control Steering : simulink/Continuous/PID Controller  Controller=PI  Form=Parallel  TimeDomain=Discrete-time  SampleTime=Ts  IntegratorMethod=Forward Euler  FilterMethod=Forward Euler  ControllerParametersSource=internal  P=0.219020351848633  I=0.4510120195392  D=0  UseFilter=on  N=100  TunerSelectOption=Transfer Function Based (PID Tuner App)  InitialConditionSource=internal  InitialConditionForIntegrator=0  InitialConditionForFilter=0  DifferentiatorICPrevScaledInput=0  ExternalReset=none  TrackingMode=off  Kt=1  LimitOutput=off  UpperSaturationLimit=inf  LowerSaturationLimit=-inf  LinearizeAsGain=on  AntiWindupMode=none  Kb=1  POutMin=[]  POutMax=[]  IOutMin=[]  IOutMax=[]  DOutMin=[]  DOutMax=[]  NOutMin=[]  NOutMax=[]  SumOutMin=[]  SumOutMax=[]  SaturationOutMin=[]  SaturationOutMax=[]  PParamMin=[]  PParamMax=[]  IParamMin=[]  IParamMax=[]  DParamMin=[]  DParamMax=[]  NParamMin=[]  NParamMax=[]  KbParamMin=[]  KbParamMax=[]  KtParamMin=[]  KtParamMax=[]  KbOutMin=[]  KbOutMax=[]  KtOutMin=[]  KtOutMax=[]  IntegratorOutMin=[]  IntegratorOutMax=[]  FilterOutMin=[]  FilterOutMax=[]  SumI1OutMin=[]  SumI1OutMax=[]  SumI2OutMin=[]  SumI2OutMax=[]  SumI3OutMin=[]  SumI3OutMax=[]  SumI4OutMin=[]  SumI4OutMax=[]  SumDOutMin=[]  SumDOutMax=[]  DifferentiatorOutMin=[]  DifferentiatorOutMax=[]  FilterDiffOutCoefMin=[]  FilterDiffOutCoefMax=[]  ReciprocalOutMin=[]  ReciprocalOutMax=[]  SumDenOutMin=[]  SumDenOutMax=[]  SumNumOutMin=[]  SumNumOutMax=[]  DivideOutMin=[]  DivideOutMax=[]  IntegratorContinuousStateAttributes=''  IntegratorStateMustResolveToSignalObject=off  IntegratorRTWStateStorageClass=Auto  FilterContinuousStateAttributes=''  FilterStateMustResolveToSignalObject=off  FilterRTWStateStorageClass=Auto  ParallelPVariant=InternalParameters  IdealPVariant=Disabled  IVariant=InternalParameters  DVariant=Disabled  IntegratorVariant=Discrete  SatVariant=Disabled  AWVariant=Passthrough  PCopyVariant=Disabled  TRVariant=Disabled  FdbkBlocksVariant=Forward  IdealPFdbkVariant=Disabled  SatFdbkVariant=Disabled  DerivativeFilterVariant=Disabled  NVariant=Disabled  NCopyVariant=Disabled_SignalSpec  FilterICVariant=Disabled  IntegratorICVariant=InternalICs  ExternalResetVariant=Disabled  TRSumVariant=Passthrough  SumFdbkVariant=Disabled  SumVariant=Sum_PI
  Sum1 : Sum  Inputs=|+-
  Steering Reference : Outport
  Controlled Output : Outport  Port=2
  wires:
  Sum1/1 -> PID Control Steering/1  "Delta Error"
  Step input/1 -> Sum1/1
  Measured Steering Angle/1 -> Gain1/1, Controlled Output/1
  PID Control Steering/1 -> Steering Reference/1
  Gain1/1 -> Sum1/2

== system bike_model_pidTuning/Physical Bike/ Addition of oscillations ==
  Roll Angle : Inport
  Steering Angle : Inport  Port=2
  Roll Rate : Inport  Port=3
  Mux : Mux  Inputs=3
  To Workspace : ToWorkspace  VariableName=states_true  SaveFormat=Timeseries  SampleTime=Ts
  To Workspace1 : ToWorkspace  VariableName=True_roll_angle  SaveFormat=Structure  SampleTime=Ts
  To Workspace2 : ToWorkspace  VariableName=True_roll_rate  SaveFormat=Structure  SampleTime=Ts
  To Workspace3 : ToWorkspace  VariableName=True_steering_angle  SaveFormat=Structure  SampleTime=-1
  True States : Outport
  wires:
  Steering Angle/1 -> To Workspace3/1, Mux/2
  Roll Rate/1 -> Mux/3, To Workspace2/1
  Roll Angle/1 -> To Workspace1/1, Mux/1  "True Roll Angle"
  Mux/1 -> True States/1, To Workspace/1

== system bike_model_pidTuning/Physical Bike/Centripetal Acceleration Calculator ==
  True Steering Angle : Inport
  True Velocity : Inport  Port=2
  Divide : Product  Inputs=*/
  Gain : Gain  Gain=sin(lambda_real)
  Multiply : Product
  Square : Math  Operator=square  SaturateOnIntegerOverflow=on
  Tan : Trigonometry  Operator=tan
  b Real Bike : Constant  Value=b_real
  Centripetal Acceleration : Outport
  wires:
  True Velocity/1 -> Square/1
  Square/1 -> Divide/1
  b Real Bike/1 -> Divide/2
  True Steering Angle/1 -> Gain/1
  Divide/1 -> Multiply/1
  Tan/1 -> Multiply/2
  Multiply/1 -> Centripetal Acceleration/1
  Gain/1 -> Tan/1

== system bike_model_pidTuning/Physical Bike/Check Phi Limits ==
  x : Inport
  Roll Lower Bound : simulink/Model Verification/Check Static  Lower Bound  Description=min_roll <= u  min=min_roll  min_included=on  enabled=on  stopWhenAssertionFail=on  export=off  icon=graphic
      settings: SourceProductName=Simulink
  Roll Upper Bound : simulink/Model Verification/Check Static  Upper Bound  Description=u <= max_roll  max=max_roll  max_included=on  enabled=on  stopWhenAssertionFail=on  export=off  icon=graphic
      settings: SourceProductName=Simulink  SourceProductBaseCode=SL
  wires:
  x/1 -> Roll Lower Bound/1, Roll Upper Bound/1  "Roll Angle"

== system bike_model_pidTuning/Physical Bike/Global Angles and Coordinates Calculator - Position ==
  note: True Steering
      | Angle
  True Velocity : Inport
  True Steering Angle : Inport  Port=2
  Gain1 : Gain  Gain=sin(lambda_compFilter)
  Measured Bike Angles to Global Angles : Subsystem
  Measured Global Angles to Global Coordinates : Subsystem
  Sum : Sum  Inputs=++|
  True Position : Outport
  True Heading : Outport  Port=2
  wires:
  Measured Bike Angles to Global Angles/1(Psi) -> Sum/2, Measured Global Angles to Global Coordinates/2(Psi)
  Gain1/1 -> Measured Bike Angles to Global Angles/2(Measured Steering Angle)
  Sum/1 -> True Heading/1
  Measured Bike Angles to Global Angles/2(Beta) -> Sum/1, Measured Global Angles to Global Coordinates/3(Beta)
  Measured Global Angles to Global Coordinates/1("Position (X, Y)") -> True Position/1
  True Velocity/1 -> Measured Global Angles to Global Coordinates/1(Velocity), Measured Bike Angles to Global Angles/1(Velocity)
  True Steering Angle/1 -> Gain1/1

== system bike_model_pidTuning/Physical Bike/Lateral Acceleration (due to Roll) Calculator ==
  Roll Acceleration : Inport
  Constant3 : Constant  Value=IMU_height_real
  Multiply : Product
  Lateral Acceleration : Outport
  wires:
  Multiply/1 -> Lateral Acceleration/1
  Constant3/1 -> Multiply/1
  Roll Acceleration/1 -> Multiply/2

== system bike_model_pidTuning/Physical Bike/Path Plotter Reality ==
  Position : Inport
  Demux : Demux  Outputs=2
  To Workspace : ToWorkspace  VariableName=X_BIKE  SaveFormat=Timeseries  SampleTime=Ts
  To Workspace1 : ToWorkspace  VariableName=Y_BIKE  SaveFormat=Timeseries  SampleTime=Ts
  XY Graph : simulink/Sinks/XY Graph  Commented=on  xmin=min(path_x)-5  xmax=max(path_x)+5  ymin=min(path_y)-5  ymax=max(path_y)+5  st=-1
  wires:
  Demux/1 -> XY Graph/1, To Workspace/1  "X"
  Demux/2 -> XY Graph/2, To Workspace1/1  "Y"
  Position/1 -> Demux/1

== system bike_model_pidTuning/Reference Position /Reference Position and Angle Selector ==
  total travelled distance : Inport
  1-D Lookup Table : Lookup_n-D  NumberOfTableDimensions=1  BreakpointsForDimension1=cumulative_dist_along_path  Table=path_x  ExtrapMethod=Clip  DiagnosticForOutOfRangeInput=Error  InternalRulePriority=Speed  RndMeth=Simplest  InputSameDT=on
  1-D Lookup Table1 : Lookup_n-D  NumberOfTableDimensions=1  BreakpointsForDimension1=cumulative_dist_along_path  Table=path_y  ExtrapMethod=Clip  DiagnosticForOutOfRangeInput=Error  InternalRulePriority=Speed  RndMeth=Simplest  InputSameDT=on
  Atan2 : Trigonometry  Operator=atan2
  Derivative : Derivative
  Derivative1 : Derivative
  Scope : Scope
  Unwrap : dspsigops/Unwrap  tol=pi  InputProcessing=Columns as channels (frame based)  running=off
  X_sigma : Outport
  Y_sigma : Outport  Port=2
  psi_sigma : Outport  Port=3
  wires:
  total travelled distance/1 -> 1-D Lookup Table1/1, 1-D Lookup Table/1
  Unwrap/1 -> Scope/1, psi_sigma/1
  1-D Lookup Table/1 -> X_sigma/1, Derivative1/1  "interpolated path x value"
  Derivative1/1 -> Atan2/2  "dx"
  Derivative/1 -> Atan2/1  "dy"
  Atan2/1 -> Unwrap/1
  1-D Lookup Table1/1 -> Y_sigma/1, Derivative/1  "interpolated path y value"

== system bike_model_pidTuning/Reference Position /Subsystem1 ==
  total travelled distance : Inport
  1-D Lookup Table : Lookup_n-D  NumberOfTableDimensions=1  BreakpointsForDimension1=cumulative_dist_along_path  Table=path_x  ExtrapMethod=Clip  DiagnosticForOutOfRangeInput=Error  InternalRulePriority=Speed  RndMeth=Simplest  InputSameDT=on
  1-D Lookup Table1 : Lookup_n-D  NumberOfTableDimensions=1  BreakpointsForDimension1=cumulative_dist_along_path  Table=path_y  ExtrapMethod=Clip  DiagnosticForOutOfRangeInput=Error  InternalRulePriority=Speed  RndMeth=Simplest  InputSameDT=on
  Atan2 : Trigonometry  Operator=atan2
  Derivative : Derivative
  Derivative1 : Derivative
  Scope : Scope
  Unwrap : dspsigops/Unwrap  tol=pi  InputProcessing=Columns as channels (frame based)  running=off
  X_sigma : Outport
  Y_sigma : Outport  Port=2
  psi_sigma : Outport  Port=3
  wires:
  total travelled distance/1 -> 1-D Lookup Table1/1, 1-D Lookup Table/1
  Unwrap/1 -> Scope/1, psi_sigma/1
  1-D Lookup Table/1 -> X_sigma/1, Derivative1/1  "interpolated path x value"
  Derivative1/1 -> Atan2/2  "dx"
  Derivative/1 -> Atan2/1  "dy"
  Atan2/1 -> Unwrap/1
  1-D Lookup Table1/1 -> Y_sigma/1, Derivative/1  "interpolated path y value"

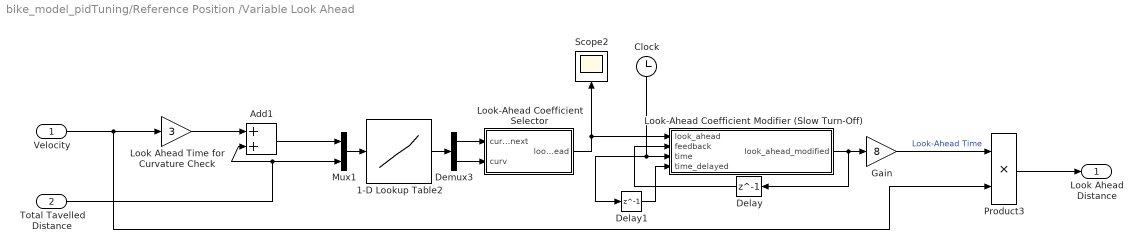
== system bike_model_pidTuning/Reference Position /Variable Look Ahead ==
  Velocity : Inport
  Total Tavelled Distance : Inport  Port=2
  1-D Lookup Table2 : Lookup_n-D  NumberOfTableDimensions=1  BreakpointsForDimension1=cumulative_dist_along_path  Table=curvature  ExtrapMethod=Clip  DiagnosticForOutOfRangeInput=Error  InternalRulePriority=Speed  RndMeth=Simplest  InputSameDT=on
  Add1 : Sum
  Clock : Clock
  Delay : Delay  DelayLength=1
  Delay1 : Delay  DelayLength=1
  Demux3 : Demux  Outputs=2
  Gain : Gain  Gain=8
  Look Ahead Time for Curvature Check : Gain  Gain=3
  Look-Ahead Coefficient Selector : MATLAB Function  TreatAsAtomicUnit=on
  "Look-Ahead Coefficient Modifier (Slow Turn-Off) " : MATLAB Function  TreatAsAtomicUnit=on
  Mux1 : Mux  Inputs=2
  Product3 : Product
  Scope2 : Scope
  Look Ahead Distance : Outport
  wires:
  Look Ahead Time for Curvature Check/1 -> Add1/1
  Delay/1 -> "Look-Ahead Coefficient Modifier (Slow Turn-Off) "/2(feedback)
  "Look-Ahead Coefficient Modifier (Slow Turn-Off) "/1(look_ahead_modified) -> Delay/1, Gain/1
  Demux3/1 -> Look-Ahead Coefficient Selector/1(curv_next)
  Look-Ahead Coefficient Selector/1(look_ahead) -> "Look-Ahead Coefficient Modifier (Slow Turn-Off) "/1(look_ahead), Scope2/1
  Clock/1 -> "Look-Ahead Coefficient Modifier (Slow Turn-Off) "/3(time), Delay1/1
  Delay1/1 -> "Look-Ahead Coefficient Modifier (Slow Turn-Off) "/4(time_delayed)
  1-D Lookup Table2/1 -> Demux3/1
  Total Tavelled Distance/1 -> Add1/2, Mux1/2
  Demux3/2 -> Look-Ahead Coefficient Selector/2(curv)
  Gain/1 -> Product3/1  "Look-Ahead Time"
  Add1/1 -> Mux1/1
  Mux1/1 -> 1-D Lookup Table2/1
  Velocity/1 -> Product3/2, Look Ahead Time for Curvature Check/1
  Product3/1 -> Look Ahead Distance/1

== system bike_model_pidTuning/Path Tracking Controller PID Tuning 2/Tuning of Direction (Heading Control)/Measured Bike Angles to Global Angles ==
  note: Verification of the equivalence of the calculus for Beta estimation
  Velocity : Inport
  Measured Steering Angle : Inport  Port=2
  Gain : Gain  Gain=1/b_compFilter
  Integrator : Integrator
  MATLAB Function : MATLAB Function  TreatAsAtomicUnit=on
  Multiply : Product
  Parameters : Constant  Value=parameters_compFilter
  Scope : Scope  NumInputPorts=2
  Tan : Trigonometry  Operator=tan
  Psi : Outport
  Beta : Outport  Port=2
  wires:
  Integrator/1 -> Psi/1
  MATLAB Function/1(psi_d) -> Scope/1, Integrator/1
  Measured Steering Angle/1 -> Tan/1, MATLAB Function/3(delta)
  Parameters/1 -> MATLAB Function/2(parameters_model)
  Velocity/1 -> Multiply/1, MATLAB Function/1(v)
  MATLAB Function/2(beta) -> Beta/1
  Tan/1 -> Multiply/2
  Multiply/1 -> Gain/1
  Gain/1 -> Scope/2

== system bike_model_pidTuning/Path Tracking Controller PID Tuning 2/Tuning of Direction (Heading Control)/Measured Global Angles to Global Coordinates ==
  Velocity : Inport
  Psi : Inport  Port=2
  Beta : Inport  Port=3
  MATLAB Function1 : MATLAB Function  TreatAsAtomicUnit=on
  Mux1 : Mux  Inputs=2
  "Velocity (Xdot, Ydot)" : Outport
  wires:
  MATLAB Function1/2(Ydot) -> Mux1/2  "Ydot"
  MATLAB Function1/1(Xdot) -> Mux1/1  "Xdot"
  Psi/1 -> MATLAB Function1/2(psi)
  Beta/1 -> MATLAB Function1/3(beta)
  Velocity/1 -> MATLAB Function1/1(v)
  Mux1/1 -> "Velocity (Xdot, Ydot)"/1

== system bike_model_pidTuning/Path Tracking Controller PID Tuning 2/Tuning of Direction (Heading Control)/Psi to Delta ==
  psi_sigma : Inport
  Gain : Gain  Gain=1/parameters_compFilter(4)
  Gain1 : Gain  Gain=parameters_compFilter(3)
  Gain2 : Gain  Gain=input_velocity*parameters_compFilter(3)/parameters_compFilter(4)
  Integrator : Integrator
  MATLAB Function : MATLAB Function  TreatAsAtomicUnit=on
  Sum : Sum  Inputs=+-
  delta : Outport
  wires:
  Gain/1 -> delta/1
  Sum/1 -> Gain/1
  Gain1/1 -> Sum/1
  psi_sigma/1 -> MATLAB Function/1(psi_sigma), Gain1/1
  Gain2/1 -> Sum/2
  Integrator/1 -> Gain2/1
  MATLAB Function/1(y) -> Integrator/1

== system bike_model_pidTuning/Path Tracking Controller PID Tuning 2/Tuning of Lateral Position Control/Lateral Error ==
  Psi Sigma : Inport
  Position Error (X,Y) : Inport  Port=2
  Cos : Trigonometry  Operator=cos
  Demux : Demux  Outputs=2
  Product : Product
  Product1 : Product
  Sin : Trigonometry
  Sum : Sum  Inputs=+-|
  To Workspace1 : ToWorkspace  VariableName=X_ERR  SaveFormat=Timeseries  SampleTime=Ts
  To Workspace2 : ToWorkspace  VariableName=Y_ERR  SaveFormat=Timeseries  SampleTime=Ts
  To Workspace4 : ToWorkspace  VariableName=LAT_ERR  SaveFormat=Timeseries  SampleTime=Ts
  Lateral Error : Outport
  wires:
  Cos/1 -> Product/2
  Sin/1 -> Product1/1
  Psi Sigma/1 -> Cos/1, Sin/1
  Product/1 -> Sum/1
  Sum/1 -> To Workspace4/1, Lateral Error/1  "Lateral Error"
  Demux/1 -> To Workspace2/1, Product1/2  "X Position Error"
  Demux/2 -> To Workspace1/1, Product/1  "Y Position Error"
  Position Error (X,Y)/1 -> Demux/1
  Product1/1 -> Sum/2
